simulink model "E5_3_Harmonicas"  (R2018a)
settings: Solver=VariableStepAuto  StartTime=0.0  StopTime=2  RelTol=1e-3
libraries: powerlib x15, powerlib_meascontrol x1
settings Model: Creator=Rafael Pavan  LastModifiedBy=Rafael Pavan
settings SolverCC: ZeroCrossAlgorithm=Adaptive
settings DebuggingCC: MaxConsecutiveZCsMsg=none

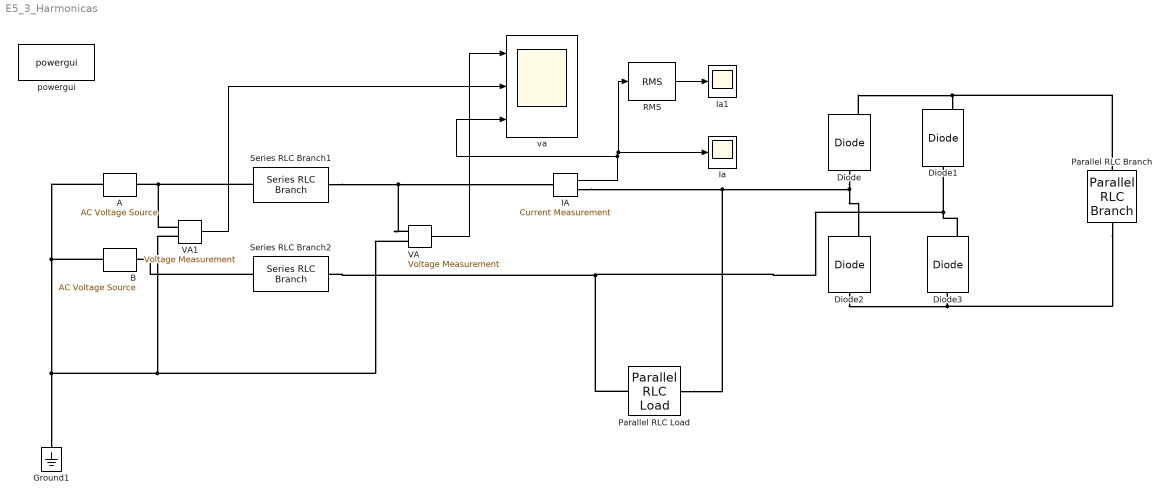
== system E5_3_Harmonicas ==
  A : powerlib/Electrical Sources/AC Voltage Source  Amplitude=179.605  Phase=0  Frequency=60  SampleTime=0  Measurements=None  BusType=PV  Pref=100e4  Qref=0  Qmin=-inf  Qmax=+inf
  B : powerlib/Electrical Sources/AC Voltage Source  Amplitude=179.605  Phase=-120  Frequency=60  SampleTime=0  Measurements=None  BusType=PV  Pref=100e4  Qref=0  Qmin=-inf  Qmax=+inf
  Diode{,1..3} (4 alike) : powerlib/Power Electronics/Diode  Ron=0.001  Lon=0  Vf=0.8  IC=0  UseSnubber=0  Rs=500  Cs=250e-9  Measurements=on
  Ground1 : powerlib/Elements/Ground  LConnTagsString=a
  IA : powerlib/Measurements/Current Measurement  PhasorSimulation=off  OutputType=Complex  PSBequivalent=0
  Ia : Scope
  Ia1 : Scope
  Parallel RLC Branch : powerlib/Elements/Parallel RLC Branch  LConnTagsString=a  RConnTagsString=__new0  BranchType=RC  Resistance=50  Inductance=100e-3  SetiL0=off  InitialCurrent=0  Capacitance=200e-6  Setx0=off  InitialVoltage=0  Measurements=None
  Parallel RLC Load : powerlib/Elements/Parallel RLC Load  LConnTagsString=a  RConnTagsString=__new0  NominalVoltage=220  NominalFrequency=60  ActivePower=12e3  InductivePower=0  CapacitivePower=0  Setx0=off  InitialVoltage=0  SetiL0=off  InitialCurrent=0  Measurements=None  LoadType=constant Z
      settings: AttributesFormatString=\n  SourceProductName=Simscape Power Systems  SourceProductBaseCode=PS
  RMS : powerlib_meascontrol/Measurements/RMS  TrueRMS=on  Freq=60  RMSInit=120  Ts=0
  Series RLC Branch1 : powerlib/Elements/Series RLC Branch  LConnTagsString=__new0  RConnTagsString=__new0  BranchType=L  Resistance=0.1  Inductance=6.631e-5  SetiL0=off  InitialCurrent=0  Capacitance=500e-6  Setx0=off  InitialVoltage=0  Measurements=None
  Series RLC Branch2 : powerlib/Elements/Series RLC Branch  LConnTagsString=__new0  RConnTagsString=__new0  BranchType=L  Resistance=0.1  Inductance=6.631e-5  SetiL0=off  InitialCurrent=0  Capacitance=3  Setx0=off  InitialVoltage=0  Measurements=None
  VA : powerlib/Measurements/Voltage Measurement  PhasorSimulation=off  OutputType=Complex  PSBequivalent=0
  VA1 : powerlib/Measurements/Voltage Measurement  PhasorSimulation=off  OutputType=Complex  PSBequivalent=0
  powergui : powerlib/powergui  Priority=1  SimulationMode=Continuous  SampleTime=50e-6  frequency=60  Iterations=50  frequencyindice=60  Pbase=100e6  ErrMax=1e-4  UnitsV=kV  UnitsW=MW  buscounter=0  FunctionMessages=on  echomessages=off  EnableUseOfTLC=off  CurrentSourceSwitches=off  DisableSnubberDevices=off  DisableRonSwitches=off  DisableVfSwitches=off  DisplayEquations=off  SolverType=Tustin/Backward Euler (TBE)  Interpol=off  ExternalGateDelay=off  methode=off  Ts=100  x0status=blocks  SPID=on  SwTol=0  HookPort=off  RestoreLinks=warning  ResistiveCurrentMeasurement=off  Frange=[0:2:500]  Ylog=off  Xlog=on  ShowGrid=off  save=off  variable=ZData  structure=va  ZoomFFT=off  StartTime=0.2  cycles=12  DisplayStyle=1  fundamental=60  FreqAxis=off  MaxFrequency=3000  frequencyindicesteady=1  RmsSteady=2  display=off
  va : Scope  NumInputPorts=3
  wires:
  IA/1 -> va/3, RMS/1, Ia/1
  VA/1 -> va/1
  RMS/1 -> Ia1/1
  VA1/1 -> va/2
  connections:
  Series RLC Branch1/RConn1 -- VA1/LConn1 -- A/RConn1
  Series RLC Branch2/RConn1 -- B/RConn1
  Series RLC Branch1/LConn1 -- VA/LConn1 -- IA/LConn1
  Diode2/LConn1 -- Parallel RLC Branch/RConn1 -- Diode3/LConn1
  B/LConn1 -- A/LConn1 -- VA1/LConn2 -- VA/LConn2 -- Ground1/LConn1
  Diode/RConn1 -- Parallel RLC Branch/LConn1 -- Diode1/RConn1
  IA/RConn1 -- Parallel RLC Load/RConn1 -- Diode/LConn1 -- Diode2/RConn1
  Diode3/RConn1 -- Diode1/LConn1 -- Parallel RLC Load/LConn1 -- Series RLC Branch2/LConn1
